simulink model "automatic_transmission"  (R2018a)
settings: Solver=ode5  StartTime=0.0  StopTime=30  FixedStep=0.04  RelTol=1e-3
undefined symbols (not defined in the file or in its folder): A, cd, DOWN_TABLE, DOWN_TH_BP, EMAP, FDR, fr, g, grade, Jei, Jveh, kFactor, m, NE_VEC, R, rho, sigbuilder_block, SpeedRatio, TH_VEC, TorqueRatio, UP_TABLE, UP_TH_BP
settings Model: Creator=Saurabh Suman  LastModifiedBy=Saurabh Suman

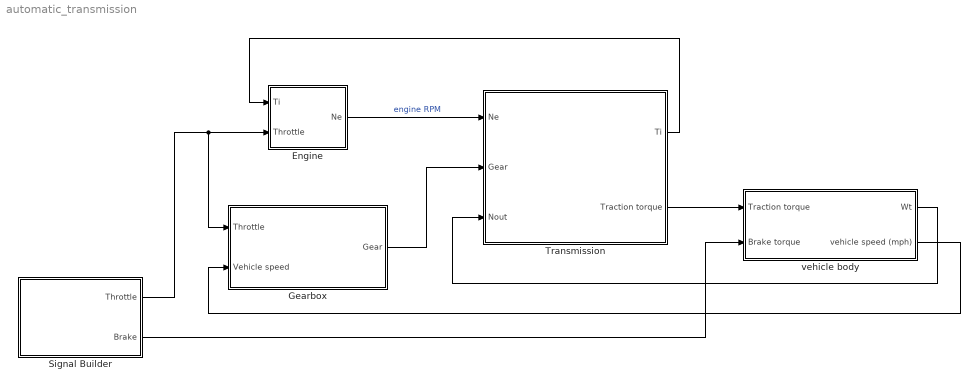
== system automatic_transmission ==
  Engine : Subsystem
  Gearbox : Subsystem
  Signal Builder : Subsystem  Tag=STV Subsys  LoadFcn=sigbuilder_block('load');  StartFcn=sigbuilder_block('start');  StopFcn=sigbuilder_block('stop');  ClipboardFcn=sigbuilder_block('clipboard');  mask(Sigbuilder block){tuvar=[0:10]}
      mask help: Simulink:masks:SigbuilderBlock_MD
      mask init:
      | if ~strcmp(get_param(bdroot(gcbh),'SimulationStatus'),'stopped') tuvar = sigbuilder_block('maskInit'); end
      settings: CopyFcn=sigbuilder_block('copy');  DeleteFcn=sigbuilder_block('delete');  ModelCloseFcn=sigbuilder_block('modelClose');  PreSaveFcn=sigbuilder_block('preSave');  PauseFcn=sigbuilder_block('pause');  ContinueFcn=sigbuilder_block('continue');  NameChangeFcn=sigbuilder_block('namechange');  OpenFcn=sigbuilder_block('open',[448.8 179.4 550.8 400.2 ]);  CloseFcn=sigbuilder_block('close');
      mask Display: plot(0, 0, 100, 100,[2, 2, 32, 32, 2], [68, 8, 8, 68, 68],[32, 2], [38, 38], [32, 19, 2],[53, 60, 44], [32, 17, 17, 2],[16, 16, 31, 31]);txt = getActiveGroup(gcbh);text(2, 100, txt,'verticalAlignment', 'top');
  Transmission : Subsystem
  vehicle body : Subsystem
  wires:
  Signal Builder/1(Throttle) -> Engine/2(Throttle), Gearbox/1(Throttle)
  Engine/1(Ne) -> Transmission/1(Ne)  "engine RPM"
  Gearbox/1(Gear) -> Transmission/2(Gear)
  Transmission/1(Ti) -> Engine/1(Ti)
  vehicle body/2(vehicle speed (mph)) -> Gearbox/2(Vehicle speed)
  vehicle body/1(Wt) -> Transmission/3(Nout)
  Signal Builder/2(Brake) -> vehicle body/2(Brake torque)
  Transmission/2(Traction torque) -> vehicle body/1(Traction torque)

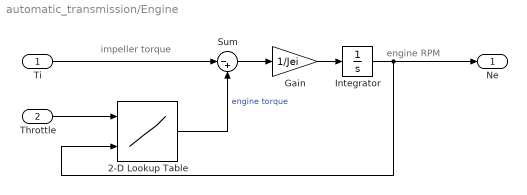
== system automatic_transmission/Engine ==
  note: engine RPM
  note: impeller torque
  Ti : Inport
  Throttle : Inport  Port=2
  2-D Lookup Table : Lookup_n-D  BreakpointsForDimension1=TH_VEC  BreakpointsForDimension2=NE_VEC  Table=EMAP  InternalRulePriority=Speed  RndMeth=Simplest  InputSameDT=on
  Gain : Gain  Gain=1/Jei
  Integrator : Integrator  InitialCondition=1000  LimitOutput=on  UpperSaturationLimit=6000  LowerSaturationLimit=600
  Sum : Sum  Inputs=|-+
  Ne : Outport
  wires:
  Sum/1 -> Gain/1
  Gain/1 -> Integrator/1
  Integrator/1 -> Ne/1, 2-D Lookup Table/2
  Throttle/1 -> 2-D Lookup Table/1
  Ti/1 -> Sum/1
  2-D Lookup Table/1 -> Sum/2  "engine torque"

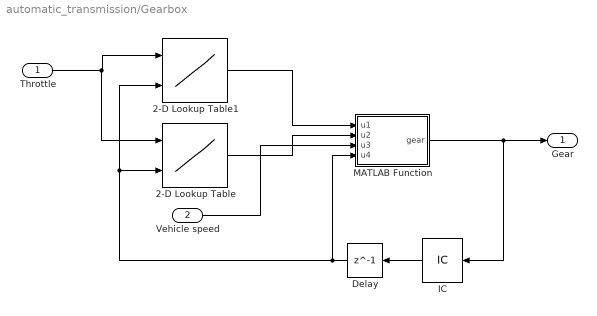
== system automatic_transmission/Gearbox ==
  Throttle : Inport
  Vehicle speed : Inport  Port=2
  2-D Lookup Table : Lookup_n-D  BreakpointsForDimension1=DOWN_TH_BP  BreakpointsForDimension2=[1:4]  Table=DOWN_TABLE  InternalRulePriority=Speed  RndMeth=Simplest  InputSameDT=on
  2-D Lookup Table1 : Lookup_n-D  BreakpointsForDimension1=UP_TH_BP  BreakpointsForDimension2=[1:4]  Table=UP_TABLE  InternalRulePriority=Speed  RndMeth=Simplest  InputSameDT=on
  Delay : Delay  DelayLength=1  InitialCondition=0
  IC : InitialCondition
  MATLAB Function : MATLAB Function  TreatAsAtomicUnit=on
  Gear : Outport
  wires:
  Delay/1 -> 2-D Lookup Table/2, 2-D Lookup Table1/2, MATLAB Function/4(u4)
  Vehicle speed/1 -> MATLAB Function/3(u3)
  MATLAB Function/1(gear) -> Gear/1, IC/1
  2-D Lookup Table1/1 -> MATLAB Function/1(u1)
  Throttle/1 -> 2-D Lookup Table/1, 2-D Lookup Table1/1
  2-D Lookup Table/1 -> MATLAB Function/2(u2)
  IC/1 -> Delay/1

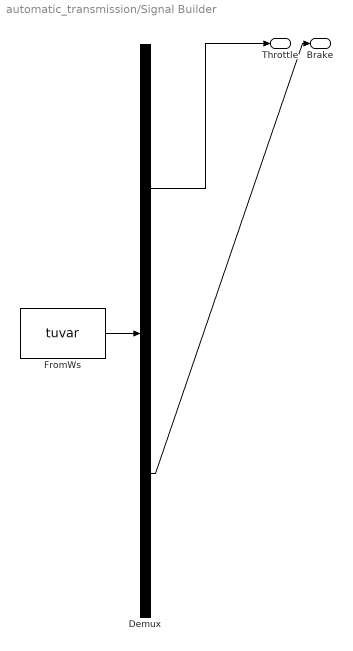
== system automatic_transmission/Signal Builder ==
  Demux : Demux  Tag=STV Demux  Outputs=2
  FromWs : FromWorkspace  Tag=STV FromWs  VariableName=tuvar  SampleTime=0
      SigBuilderData=|
      | common.afterFinalStr = 'Extrapolate'
      | common.sampleTime = 0
      | dataSet(1).timeRange = [0 50]
      | dataSet(1).name = 'Passing Maneuver'
      | dataSet(2).timeRange = [0 50]
      | dataSet(2).name = 'Gardual Acceleration'
      | dataSet(3).timeRange = [0 50]
      | dataSet(3).name = 'Hard Braking'
      | dataSet(4).timeRange = [0 50]
      | dataSet(4).name = 'Coasting'
      | sbobj.Groups(1).Name = 'Passing Maneuver'
      | sbobj.Groups(1).Signals(1).Name = 'Throttle'
      | sbobj.Groups(1).Signals(1).XData = [0 14.9 15 50]
      | sbobj.Groups(1).Signals(1).YData = [60 40 100 60]
      | sbobj.Groups(1).Signals(2).Name = 'Brake'
      | sbobj.Groups(1).Signals(2).XData = [0 50]
      | sbobj.Groups(1).Signals(2).YData = [0 0]
      | sbobj.Groups(1).TimeRange = [0 50]
      | sbobj.Groups(2).Name = 'Gardual Acceleration'
      | sbobj.Groups(2).Signals(1).Name = 'Throttle'
      | sbobj.Groups(2).Signals(1).XData = [0 50]
      | sbobj.Groups(2).Signals(1).YData = [13.4 24]
      | sbobj.Groups(2).Signals(2).Name = 'Brake'
      | sbobj.Groups(2).Signals(2).XData = [0 50]
      | sbobj.Groups(2).Signals(2).YData = [0 0]
      | sbobj.Groups(2).TimeRange = [0 50]
      | sbobj.Groups(3).Name = 'Hard Braking'
      | sbobj.Groups(3).Signals(1).Name = 'Throttle'
      | sbobj.Groups(3).Signals(1).XData = [0 5.1 5.1 50]
      | sbobj.Groups(3).Signals(1).YData = [50 50 1 1]
      | sbobj.Groups(3).Signals(2).Name = 'Brake'
      | sbobj.Groups(3).Signals(2).XData = [0 10 10 50]
      | sbobj.Groups(3).Signals(2).YData = [0 0 325 325]
      | sbobj.Groups(3).TimeRange = [0 50]
      | sbobj.Groups(4).Name = 'Coasting'
      | sbobj.Groups(4).Signals(1).Name = 'Throttle'
      | sbobj.Groups(4).Signals(1).XData = [0 4.8 4.8 50]
      | sbobj.Groups(4).Signals(1).YData = [80 80 1 1]
      | sbobj.Groups(4).Signals(2).Name = 'Brake'
      | sbobj.Groups(4).Signals(2).XData = [0 50]
      | sbobj.Groups(4).Signals(2).YData = [0 0]
      | sbobj.Groups(4).TimeRange = [0 50]
  Throttle : Outport  Tag=STV Outport
  Brake : Outport  Tag=STV Outport  Port=2
  wires:
  Demux/1 -> Throttle/1
  FromWs/1 -> Demux/1
  Demux/2 -> Brake/1

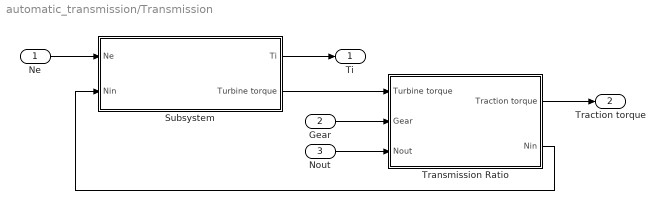
== system automatic_transmission/Transmission ==
  Ne : Inport
  Gear : Inport  Port=2
  Nout : Inport  Port=3
  Subsystem : Subsystem
  Transmission Ratio : Subsystem
  Ti : Outport
  Traction torque : Outport  Port=2
  wires:
  Ne/1 -> Subsystem/1(Ne)
  Transmission Ratio/2(Nin) -> Subsystem/2(Nin)
  Subsystem/1(Ti) -> Ti/1
  Transmission Ratio/1(Traction torque) -> Traction torque/1
  Subsystem/2(Turbine torque) -> Transmission Ratio/1(Turbine torque)
  Gear/1 -> Transmission Ratio/2(Gear)
  Nout/1 -> Transmission Ratio/3(Nout)

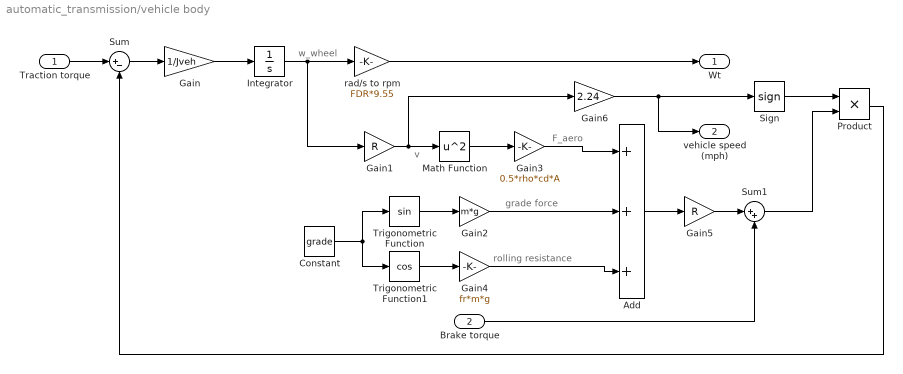
== system automatic_transmission/vehicle body ==
  note: v
  note: grade force
  note: rolling resistance
  note: F_aero
  note: w_wheel
  Traction torque : Inport
  Brake torque : Inport  Port=2
  Add : Sum  Inputs=+++
  Constant : Constant  Value=grade
  Gain : Gain  Gain=1/Jveh
  Gain1 : Gain  Gain=R
  Gain2 : Gain  Gain=m*g
  Gain3 : Gain  Gain=0.5*rho*cd*A
  Gain4 : Gain  Gain=fr*m*g
  Gain5 : Gain  Gain=R
  Gain6 : Gain  Gain=2.24
  Integrator : Integrator
  Math Function : Math  Operator=square  SaturateOnIntegerOverflow=on
  Product : Product
  Sign : Signum
  Sum : Sum  Inputs=|+-
  Sum1 : Sum  Inputs=|++
  Trigonometric Function : Trigonometry
  Trigonometric Function1 : Trigonometry  Operator=cos
  rad/s to rpm : Gain  Gain=FDR*9.55
  Wt : Outport
  vehicle speed (mph) : Outport  Port=2
  wires:
  Gain/1 -> Integrator/1
  Traction torque/1 -> Sum/1
  Integrator/1 -> Gain1/1, rad/s to rpm/1
  Add/1 -> Gain5/1
  Gain6/1 -> vehicle speed (mph)/1, Sign/1
  Sum1/1 -> Product/2
  rad/s to rpm/1 -> Wt/1
  Product/1 -> Sum/2
  Sum/1 -> Gain/1
  Trigonometric Function1/1 -> Gain4/1
  Brake torque/1 -> Sum1/2
  Gain2/1 -> Add/2
  Constant/1 -> Trigonometric Function1/1, Trigonometric Function/1
  Gain3/1 -> Add/1
  Gain4/1 -> Add/3
  Gain1/1 -> Gain6/1, Math Function/1
  Gain5/1 -> Sum1/1
  Math Function/1 -> Gain3/1
  Trigonometric Function/1 -> Gain2/1
  Sign/1 -> Product/1

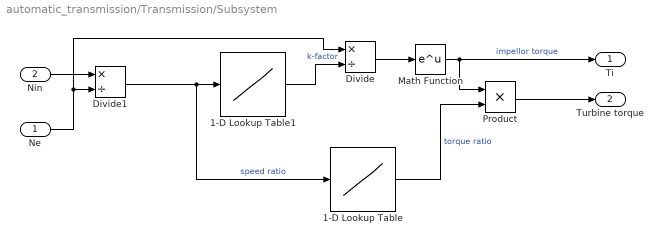
== system automatic_transmission/Transmission/Subsystem ==
  Ne : Inport
  Nin : Inport  Port=2
  1-D Lookup Table : Lookup_n-D  NumberOfTableDimensions=1  BreakpointsForDimension1=SpeedRatio  Table=TorqueRatio  InternalRulePriority=Speed  RndMeth=Simplest  InputSameDT=on
  1-D Lookup Table1 : Lookup_n-D  NumberOfTableDimensions=1  BreakpointsForDimension1=SpeedRatio  Table=kFactor  InternalRulePriority=Speed  RndMeth=Simplest  InputSameDT=on
  Divide : Product  Inputs=*/
  Divide1 : Product  Inputs=*/
  Math Function : Math  SaturateOnIntegerOverflow=on
  Product : Product
  Ti : Outport
  Turbine torque : Outport  Port=2
  wires:
  Divide1/1 -> 1-D Lookup Table/1, 1-D Lookup Table1/1  "speed ratio"
  Math Function/1 -> Ti/1, Product/1  "impellor torque"
  1-D Lookup Table/1 -> Product/2  "torque ratio"
  Divide/1 -> Math Function/1
  1-D Lookup Table1/1 -> Divide/2  "k-factor"
  Product/1 -> Turbine torque/1
  Nin/1 -> Divide1/1
  Ne/1 -> Divide/1, Divide1/2

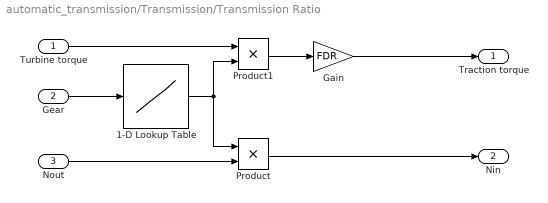
== system automatic_transmission/Transmission/Transmission Ratio ==
  Turbine torque : Inport
  Gear : Inport  Port=2
  Nout : Inport  Port=3
  1-D Lookup Table : Lookup_n-D  NumberOfTableDimensions=1  BreakpointsForDimension1=[1:4]  Table=[2.393 1.450 1.000 0.677]  InternalRulePriority=Speed  RndMeth=Simplest  InputSameDT=on
  Gain : Gain  Gain=FDR
  Product : Product
  Product1 : Product
  Traction torque : Outport
  Nin : Outport  Port=2
  wires:
  Turbine torque/1 -> Product1/1
  Product/1 -> Nin/1
  Gain/1 -> Traction torque/1
  Gear/1 -> 1-D Lookup Table/1
  1-D Lookup Table/1 -> Product/1, Product1/2
  Product1/1 -> Gain/1
  Nout/1 -> Product/2

== matlab function automatic_transmission/Gearbox/MATLAB Function ==
  data: u1 input; gear output; u2 input; u3 input; u4 input
function gear = fcn(u1,u2,u3,u4)
state=0;
if (u3>u1)
    state=1;
    if (u3>=u1)
        if(u4==4)
            u4=4;
        else
            u4=u4+1;
        end
        state=0;
    else
        state=0;
    end
elseif (u3<u2)
    state=-1;
    if(u3<=u2)
        if(u4==1)
        u4=1;
        else
        u4=u4-1;
        end
        state=0;
    else
    state=0;
    end
end
gear=u4;
